simulink model "a9"  (R2021a)
settings: Solver=VariableStepAuto  StartTime=0.0  StopTime=3  RelTol=1e-3
undefined symbols (not defined in the file or in its folder): Down, Ion, Lithium, Up
libraries: spsCurrentMeasurementLib x22, spsVoltageMeasurementLib x17, spsSeriesRLCBranchLib x11, spsGroundLib x6, powerlib_extras x4, spsACVoltageSourceLib x3, spsIGBTDiodeLib x3, dspsigops x3, spsPower3phInstantaneousLib x3, spsDiodeLib x2, spsUniversalBridgeLib x2, spsBatteryLib x1
(part 2 of 2)

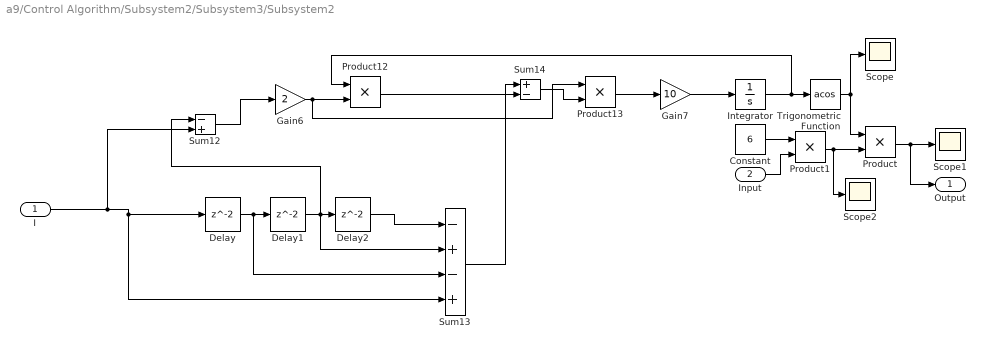
== system a9/Control Algorithm/Subsystem2/Subsystem3/Subsystem2 ==
  I : Inport
  Input : Inport  Port=2
  Constant : Constant  Value=6
  Delay : Delay
  Delay1 : Delay
  Delay2 : Delay
  Gain6 : Gain  Gain=2
  Gain7 : Gain  Gain=10
  Integrator : Integrator
  Product{,1,12..13} (4 alike) : Product
  Scope : Scope
  Scope1 : Scope
  Scope2 : Scope
  Sum12 : Sum  Inputs=-+
  Sum13 : Sum  Inputs=-+-+
  Sum14 : Sum  Inputs=+-
  Trigonometric Function : Trigonometry  Operator=acos  RemoveProtectionAgainstOutOfRangeInput=on
  Output : Outport
  wires:
  I/1 -> Sum13/4, Delay/1, Sum12/2
  Sum13/1 -> Sum14/1
  Sum14/1 -> Product13/2
  Gain6/1 -> Product13/1, Product12/2
  Delay2/1 -> Sum13/1
  Product12/1 -> Sum14/2
  Integrator/1 -> Product12/1, Trigonometric Function/1
  Delay/1 -> Sum13/3, Delay1/1
  Gain7/1 -> Integrator/1
  Sum12/1 -> Gain6/1
  Product13/1 -> Gain7/1
  Delay1/1 -> Sum12/1, Sum13/2, Delay2/1
  Product1/1 -> Scope2/1, Product/2
  Product/1 -> Output/1, Scope1/1
  Constant/1 -> Product1/1
  Input/1 -> Product1/2
  Trigonometric Function/1 -> Product/1, Scope/1

== matlab function a9/PnO MPPT ==
  settings: updateMethod=DISCRETE
  data: v input; d output; i input
function d = fcn(v,i)
persistent vprev;
persistent dprev;
persistent pprev;


   if isempty(vprev)
       vprev=0;
   end
   if isempty(dprev)
       dprev=0;
   end
   if isempty(pprev)
       pprev=0;
   end

   d = dprev;
   p = v*i;
   deltav = v - vprev;
   deltap = p -pprev;
   if deltap>0
       if deltav>0
           d = dprev - 0.05;
       elseif deltav <0
           d = dprev+0.05;
       end
   elseif deltap<0
       if deltav>0
           d = dprev+0.05;
       elseif deltav<0
           d = dprev-0.05;
       end
   end


   if d>0.9
       d=0.9;
   elseif d<0
       d=0;
   end
   vprev = v;
   pprev = p;
   dprev = d;
